simulink model "simulAMR_stateflow_indoor"  (R2024a)
settings: Solver=ode1  StartTime=0.0  StopTime=tfinal  FixedStep=tstep  MaxStep=tstep  RelTol=1e-3
values from neighbouring files (symbols this model uses):
  vehicle_wheelbase = 1    [TricycleModel.m]
undefined symbols (not defined in the file or in its folder): L, num_of_wps, T, tstep
libraries: simulink_extras x2, simulink x2
settings Model: Creator=ander  LastModifiedBy=matlab.cut

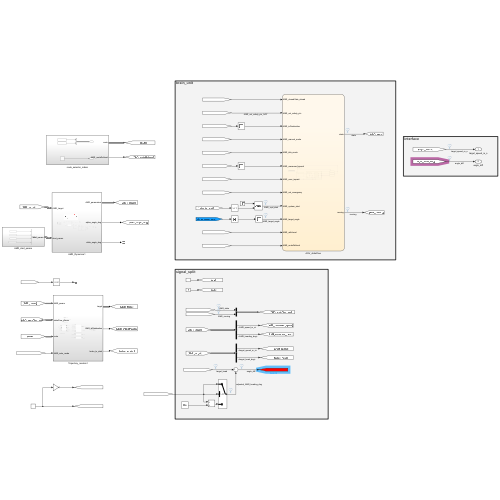
[thumbnail: Simulink's stored preview of the top-level diagram]
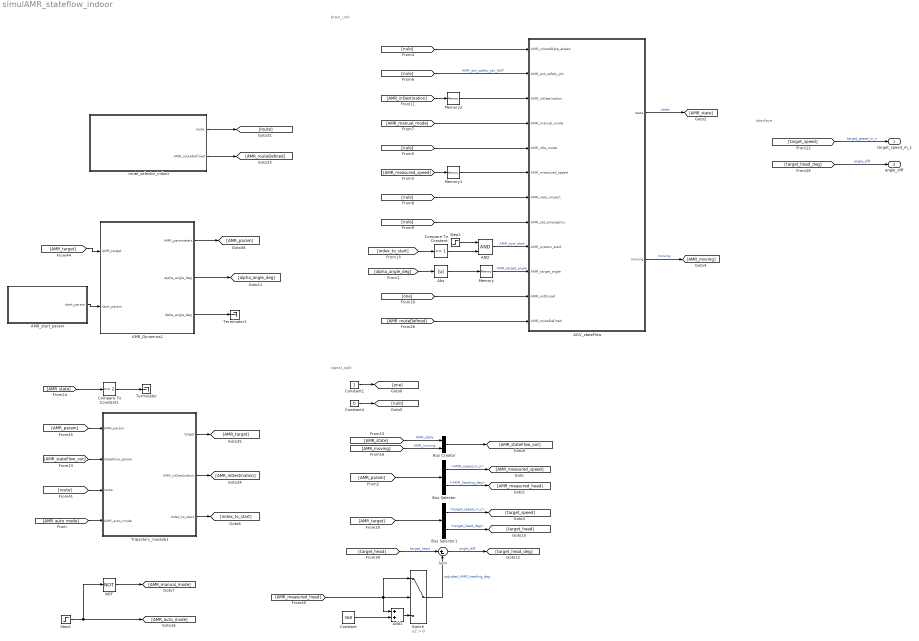
== system simulAMR_stateflow_indoor ==
  note: brain_unit
  note: interface
  note: signal_split
  AGV_stateFlow : Stateflow chart  TreatAsAtomicUnit=on
  AMR_Dynamics1 : Subsystem
  AMR_start_param : Subsystem
  AND : Logic  AllPortsSameDT=off  OutDataTypeStr=boolean
  Abs : Abs  SaturateOnIntegerOverflow=off
  Add1 : Sum
  Bus Creator : BusCreator  Inputs=2
  Bus Selector : BusSelector  OutputSignals=AMR_speed_m_s,AMR_heading_deg
  Bus Selector1 : BusSelector  OutputSignals=target_speed_m_s,target_head_deg
  Compare To Constant : simulink/Logic and Bit Operations/Compare To Constant  relop=>=  const=1  OutDataTypeStr=boolean
  Compare To Constant1 : simulink/Logic and Bit Operations/Compare To Constant  relop===  const=2  OutDataTypeStr=boolean
  Constant : Constant  Value=360
  Constant1 : Constant
  Constant4 : Constant  Value=0
  Memory : Memory
  Memory1 : Memory
  Memory2 : Memory
  NOT : Logic  Operator=NOT  IconShape=distinctive  AllPortsSameDT=off  OutDataTypeStr=boolean
  Step1 : Step  Time=20  SampleTime=tstep
  Step2 : Step  Time=10  SampleTime=0
  Sum : Sum  Inputs=|+-
  Switch : Switch  Criteria=u2 > Threshold  SaturateOnIntegerOverflow=off  InputSameDT=off
  Terminator : Terminator
  Terminator1 : Terminator
  Trajectory_module1 : Subsystem
  route_selector_indoor : Subsystem
  target_speed_m_s : Outport
  angle_diff : Outport  Port=2
  wires:
  Trajectory_module1/1(target) -> [AMR_target]
  route_selector_indoor/1(route) -> [route]
  [AMR_param] -> Trajectory_module1/1(AMR_param)
  [AMR_routeDefined] -> AGV_stateFlow/12(AMR_routeDefined)
  [nulo] -> AGV_stateFlow/1(AMR_closedGate_ahead)
  AGV_stateFlow/2(moving) -> [AMR_moving]  "moving"
  [nulo] -> AGV_stateFlow/2(AMR_ext_safety_plc)  "AMR_ext_safety_plc_NOT"
  Memory/1 -> AGV_stateFlow/10(AMR_target_angle)  "AMR_target_angle"
  Memory1/1 -> AGV_stateFlow/6(AMR_measured_speed)
  Memory2/1 -> AGV_stateFlow/3(AMR_inDestination)
  [nulo] -> AGV_stateFlow/7(AMR_near_impact)
  AGV_stateFlow/1(state) -> [AMR_state]  "state"
  [AMR_measured_speed] -> Memory1/1
  [AMR_inDestination] -> Memory2/1
  route_selector_indoor/2(AMR_routeDefined) -> [AMR_routeDefined]
  Trajectory_module1/2(AMR_inDestination) -> [AMR_inDestination]
  AMR_Dynamics1/1(AMR_parameters) -> [AMR_param]
  [one] -> AGV_stateFlow/11(AMR_withLoad)
  [AMR_stateFlow_out] -> Trajectory_module1/2(stateFlow_param)
  [AMR_manual_mode] -> AGV_stateFlow/4(AMR_manual_mode)
  [target_head_deg] -> angle_diff/1  "angle_diff"
  [route] -> Trajectory_module1/3(route)
  [nulo] -> AGV_stateFlow/5(AMR_idle_mode)
  [AMR_state] -> Compare To Constant1/1
  [AMR_target] -> AMR_Dynamics1/1(AMR_target)
  [alpha_angle_deg] -> Abs/1
  AMR_start_param/1(start_param) -> AMR_Dynamics1/2(start_param)
  [target_speed] -> target_speed_m_s/1  "target_speed_m_s"
  [target_head] -> Sum/1  "target_head"
  Switch/1 -> Sum/2  "adjusted_AMR_heading_deg"
  Constant4/1 -> [nulo]
  [AMR_param] -> Bus Selector/1
  Bus Selector1/2 -> [target_head]  "<target_head_deg>"
  Bus Selector/2 -> [AMR_measured_head]  "<AMR_heading_deg>"
  Bus Selector1/1 -> [target_speed]  "<target_speed_m_s>"
  [AMR_target] -> Bus Selector1/1
  Constant1/1 -> [one]
  [AMR_moving] -> Bus Creator/2  "AMR_moving"
  Bus Selector/1 -> [AMR_measured_speed]  "<AMR_speed_m_s>"
  [AMR_state] -> Bus Creator/1  "AMR_state"
  Bus Creator/1 -> [AMR_stateFlow_out]
  [nulo] -> AGV_stateFlow/8(AMR_set_emergency)
  Abs/1 -> Memory/1
  Step1/1 -> NOT/1, [AMR_auto_mode]
  NOT/1 -> [AMR_manual_mode]
  [AMR_auto_mode] -> Trajectory_module1/4(AMR_auto_mode)
  Compare To Constant1/1 -> Terminator/1
  Trajectory_module1/3(Index_to_start) -> [index_to_start]
  Step2/1 -> AND/1
  [index_to_start] -> Compare To Constant/1
  AND/1 -> AGV_stateFlow/9(AMR_system_start)  "AMR_syst_start"
  Compare To Constant/1 -> AND/2
  Sum/1 -> [target_head_deg]  "angle_diff"
  [AMR_measured_head] -> Switch/1, Add1/1, Switch/2
  Constant/1 -> Add1/2
  Add1/1 -> Switch/3
  AMR_Dynamics1/2(alpha_angle_deg) -> [alpha_angle_deg]
  AMR_Dynamics1/3(delta_angle_deg) -> Terminator1/1

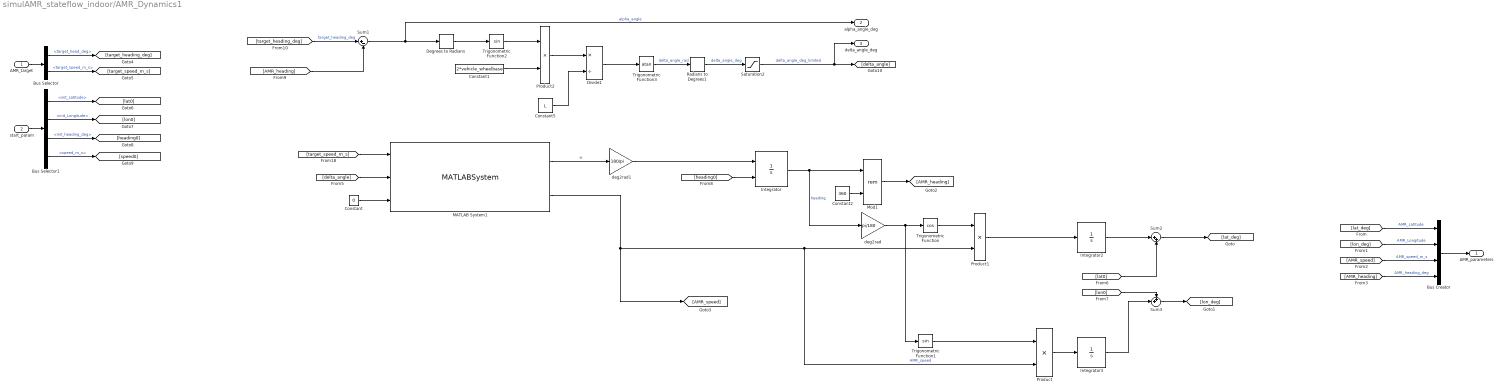
== system simulAMR_stateflow_indoor/AMR_Dynamics1 ==
  AMR_target : Inport
  start_param : Inport  Port=2
  Bus Creator : BusCreator  Inputs=4
  Bus Selector : BusSelector  OutputSignals=target_head_deg,target_speed_m_s
  Bus Selector1 : BusSelector  OutputSignals=init_Latitude,init_Longitude,init_heading_deg,speed_m_s
  Constant : Constant  Value=0
  Constant1 : Constant  Value=2*vehicle_wheelbase
  Constant2 : Constant  Value=360
  Constant5 : Constant  Value=L
  Degrees to Radians : simulink_extras/Transformations/Degrees to Radians
  Divide1 : Product  Inputs=*/
  Integrator : Integrator  InitialConditionSource=external  UpperSaturationLimit=360  LowerSaturationLimit=0
  Integrator2 : Integrator
  Integrator3 : Integrator
  MATLAB System1 : MATLABSystem  System=TricycleModel  wheel_radius=0.18  vehicle_track=0.877  vehicle_wheelbase=2.367  x0=0  y0=0  theta0=0  steering_wheel_radius=0.18  SimulateUsing=Code generation
      mask Type: TricycleModel
      mask Display:
      | disp('TricycleModel');
      | port_label('input',1,'front_wheel_speed');
      | port_label('input',2,'steering_angle');
      | port_label('input',3,'x0');
      | port_label('output',1,'angular_speed');
      | port_label('output',2,'speed');
  Mod1 : Math  Operator=rem
  Product : Product
  Product1 : Product
  Product2 : Product
  Radians to Degrees1 : simulink_extras/Transformations/Radians to Degrees
  Saturation2 : Saturate  UpperLimit=60  LowerLimit=-60
  Sum1 : Sum  Inputs=|+-
  Sum2 : Sum  Inputs=|++
  Sum3 : Sum  Inputs=++|
  Trigonometric Function : Trigonometry  Operator=cos
  Trigonometric Function1 : Trigonometry
  Trigonometric Function2 : Trigonometry
  Trigonometric Function3 : Trigonometry  Operator=atan  ApproximationMethod=CORDIC
  deg2rad : Gain  Gain=pi/180
  deg2rad1 : Gain  Gain=180/pi
  AMR_parameters : Outport
  alpha_angle_deg : Outport  Port=2
  delta_angle_deg : Outport  Port=3
  wires:
  Integrator/1 -> Mod1/1, deg2rad/1  "heading"
  MATLAB System1/2 -> [AMR_speed], Product1/2, Product/2  "AMR_speed"
  [heading0] -> Integrator/2
  deg2rad/1 -> Trigonometric Function1/1, Trigonometric Function/1
  Trigonometric Function/1 -> Product1/1
  Product1/1 -> Integrator2/1
  [lat_deg] -> Bus Creator/1  "AMR_Latitude"
  [lon_deg] -> Bus Creator/2  "AMR_Longitude"
  Bus Creator/1 -> AMR_parameters/1
  [AMR_speed] -> Bus Creator/3  "AMR_speed_m_s"
  [AMR_heading] -> Bus Creator/4  "AMR_heading_deg"
  AMR_target/1 -> Bus Selector/1
  start_param/1 -> Bus Selector1/1
  Bus Selector/1 -> [target_heading_deg]  "<target_head_deg>"
  Bus Selector/2 -> [target_speed_m_s]  "<target_speed_m_s>"
  Bus Selector1/1 -> [lat0]  "<init_Latitude>"
  Bus Selector1/2 -> [lon0]  "<init_Longitude>"
  Bus Selector1/3 -> [heading0]  "<init_heading_deg>"
  Bus Selector1/4 -> [speed0]  "<speed_m_s>"
  Product/1 -> Integrator3/1
  Trigonometric Function1/1 -> Product/1
  Sum2/1 -> [lat_deg]
  Sum3/1 -> [lon_deg]
  [lon0] -> Sum3/1
  Integrator3/1 -> Sum3/2
  MATLAB System1/1 -> deg2rad1/1  "w"
  Constant2/1 -> Mod1/2
  Mod1/1 -> [AMR_heading]
  Integrator2/1 -> Sum2/1
  [lat0] -> Sum2/2
  [target_speed_m_s] -> MATLAB System1/1
  Constant/1 -> MATLAB System1/3
  [delta_angle] -> MATLAB System1/2
  deg2rad1/1 -> Integrator/1
  [AMR_heading] -> Sum1/2
  Degrees to Radians/1 -> Trigonometric Function2/1
  Trigonometric Function2/1 -> Product2/1
  [target_heading_deg] -> Sum1/1  "target_heading_deg"
  Divide1/1 -> Trigonometric Function3/1
  Trigonometric Function3/1 -> Radians to Degrees1/1  "delta_angle_rad"
  Constant5/1 -> Divide1/2
  Product2/1 -> Divide1/1
  Constant1/1 -> Product2/2
  Sum1/1 -> alpha_angle_deg/1, Degrees to Radians/1  "alpha_angle"
  Radians to Degrees1/1 -> Saturation2/1  "delta_angle_deg"
  Saturation2/1 -> delta_angle_deg/1, [delta_angle]  "delta_angle_deg_limited"

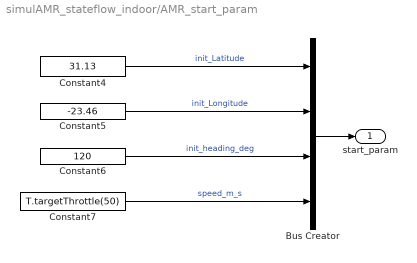
== system simulAMR_stateflow_indoor/AMR_start_param ==
  Bus Creator : BusCreator  Inputs=4
  Constant4 : Constant  Value=31.13
  Constant5 : Constant  Value=-23.46
  Constant6 : Constant  Value=120
  Constant7 : Constant  Value=T.targetThrottle(50)  VectorParams1D=off
  start_param : Outport
  wires:
  Bus Creator/1 -> start_param/1
  Constant4/1 -> Bus Creator/1  "init_Latitude"
  Constant5/1 -> Bus Creator/2  "init_Longitude"
  Constant6/1 -> Bus Creator/3  "init_heading_deg"
  Constant7/1 -> Bus Creator/4  "speed_m_s"

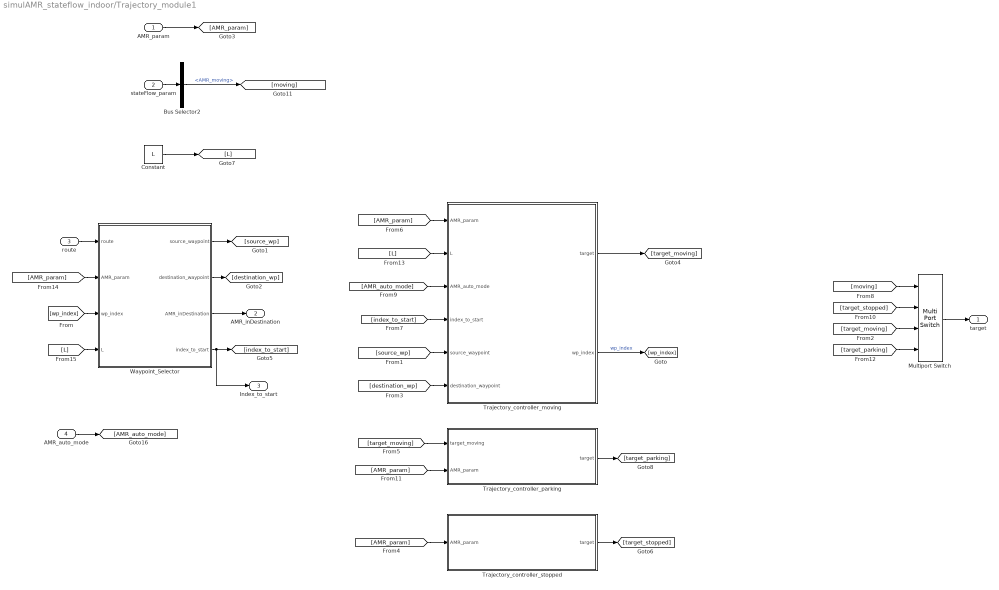
== system simulAMR_stateflow_indoor/Trajectory_module1 ==
  AMR_param : Inport
  stateFlow_param : Inport  Port=2
  route : Inport  Port=3
  AMR_auto_mode : Inport  Port=4
  Bus Selector2 : BusSelector  OutputSignals=AMR_moving
  Constant : Constant  Value=L
  Multiport Switch : MultiPortSwitch  DataPortOrder=Zero-based contiguous  zeroidx=on  SaturateOnIntegerOverflow=off  InputSameDT=off
  Trajectory_controller_moving : Subsystem
  Trajectory_controller_parking : Subsystem
  Trajectory_controller_stopped : Subsystem
  Waypoint_Selector : Subsystem
  target : Outport
  AMR_inDestination : Outport  Port=2
  Index_to_start : Outport  Port=3
  wires:
  Trajectory_controller_moving/2(wp_index) -> [wp_index]  "wp_index"
  [wp_index] -> Waypoint_Selector/3(wp_index)
  Trajectory_controller_moving/1(target) -> [target_moving]
  route/1 -> Waypoint_Selector/1(route)
  [L] -> Trajectory_controller_moving/2(L)
  Bus Selector2/1 -> [moving]  "<AMR_moving>"
  stateFlow_param/1 -> Bus Selector2/1
  [source_wp] -> Trajectory_controller_moving/5(source_waypoint)
  Waypoint_Selector/1(source_waypoint) -> [source_wp]
  Waypoint_Selector/2(destination_waypoint) -> [destination_wp]
  [destination_wp] -> Trajectory_controller_moving/6(destination_waypoint)
  AMR_param/1 -> [AMR_param]
  [AMR_param] -> Trajectory_controller_moving/1(AMR_param)
  Multiport Switch/1 -> target/1
  [moving] -> Multiport Switch/1
  [target_stopped] -> Multiport Switch/2
  [target_moving] -> Trajectory_controller_parking/1(target_moving)
  Trajectory_controller_parking/1(target) -> [target_parking]
  [AMR_param] -> Trajectory_controller_parking/2(AMR_param)
  [AMR_param] -> Trajectory_controller_stopped/1(AMR_param)
  Trajectory_controller_stopped/1(target) -> [target_stopped]
  Constant/1 -> [L]
  [AMR_param] -> Waypoint_Selector/2(AMR_param)
  [L] -> Waypoint_Selector/4(L)
  Waypoint_Selector/3(AMR_inDestination) -> AMR_inDestination/1
  [target_moving] -> Multiport Switch/3
  [target_parking] -> Multiport Switch/4
  Waypoint_Selector/4(index_to_start) -> Index_to_start/1, [index_to_start]
  [index_to_start] -> Trajectory_controller_moving/4(index_to_start)
  AMR_auto_mode/1 -> [AMR_auto_mode]
  [AMR_auto_mode] -> Trajectory_controller_moving/3(AMR_auto_mode)

== system simulAMR_stateflow_indoor/route_selector_indoor ==
  Bus Creator : BusCreator  Inputs=2
  Constant : Constant  Value=T.X
  Constant1 : Constant  Value=T.Y
  Constant2 : Constant
  route : Outport
  AMR_routeDefined : Outport  Port=2
  wires:
  Constant1/1 -> Bus Creator/2  "Y"
  Constant/1 -> Bus Creator/1  "X"
  Bus Creator/1 -> route/1  "route"
  Constant2/1 -> AMR_routeDefined/1

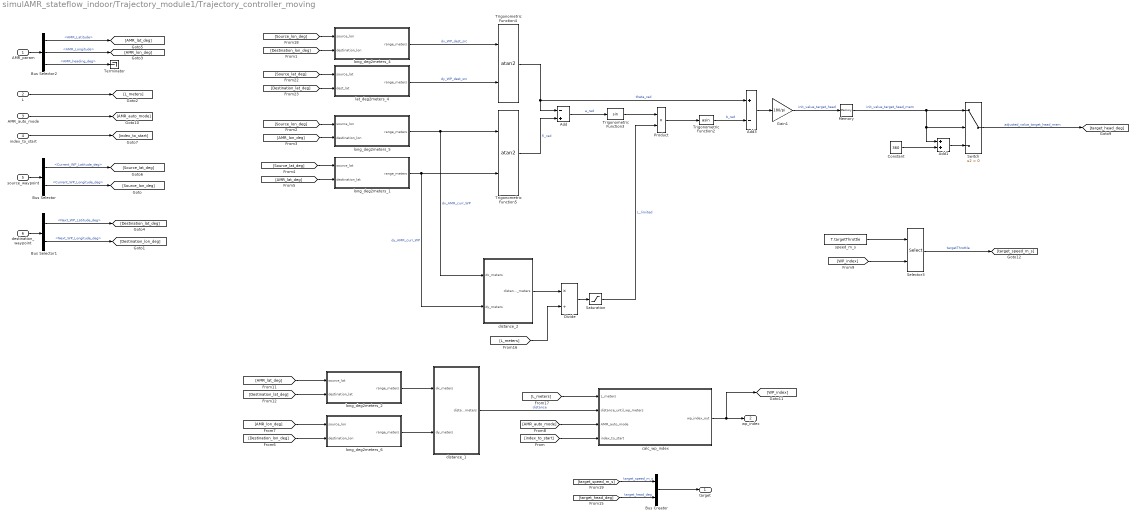
== system simulAMR_stateflow_indoor/Trajectory_module1/Trajectory_controller_moving ==
  AMR_param : Inport
  L : Inport  Port=2
  AMR_auto_mode : Inport  Port=3
  index_to_start : Inport  Port=4
  source_waypoint : Inport  Port=5
  destination_waypoint : Inport  Port=6
  Add : Sum  Inputs=-+
  Add1 : Sum
  Add3 : Sum  Inputs=+-
  Bus Creator : BusCreator  Inputs=2
  Bus Selector : BusSelector  OutputSignals=Current_WP_Latitude_deg,Current_WP_Longitude_deg
  Bus Selector1 : BusSelector  OutputSignals=Next_WP_Latitude_deg,Next_WP_Longitude_deg
  Bus Selector2 : BusSelector  OutputSignals=AMR_Latitude,AMR_Longitude,AMR_heading_deg
  Constant : Constant  Value=360
  Divide : Product  Inputs=*/
  Gain1 : Gain  Gain=180/pi
  Memory : Memory  InitialCondition=T.Yaw(1)
  Product : Product
  Saturation : Saturate  LowerLimit=0
  Selector3 : Selector  InputPortWidth=num_of_wps  IndexOptions=Index vector (port)  Indices=[1 3]  OutputSizes=1
  Switch : Switch  Criteria=u2 > Threshold  SaturateOnIntegerOverflow=off  InputSameDT=off
  Terminator : Terminator
  Trigonometric Function2 : Trigonometry  Operator=asin
  Trigonometric Function3 : Trigonometry
  Trigonometric Function4 : Trigonometry  Operator=atan2
  Trigonometric Function5 : Trigonometry  Operator=atan2
  calc_wp_index : Subsystem
  distance_1 : Subsystem  TreatAsAtomicUnit=on
  distance_2 : Subsystem  TreatAsAtomicUnit=on
  lat_deg2meters_4 : Subsystem  TreatAsAtomicUnit=on
  long_deg2meters_1 : Subsystem  TreatAsAtomicUnit=on
  long_deg2meters_2 : Subsystem  TreatAsAtomicUnit=on
  long_deg2meters_4 : Subsystem  TreatAsAtomicUnit=on
  long_deg2meters_5 : Subsystem  TreatAsAtomicUnit=on
  long_deg2meters_6 : Subsystem  TreatAsAtomicUnit=on
  speed_m_s : Constant  Value=T.targetThrottle
  target : Outport
  wp_index : Outport  Port=2
  wires:
  distance_1/1(distance_meters) -> calc_wp_index/2(distance_until_wp_meters)  "distance"
  calc_wp_index/1(wp_index_out) -> [WP_index], wp_index/1
  [Destination_lon_deg] -> long_deg2meters_6/2(destination_lon)
  Trigonometric Function4/1 -> Add3/1, Add/1  "theta_rad"
  [L_meters] -> Divide/2
  [L_meters] -> calc_wp_index/1(L_meters)
  source_waypoint/1 -> Bus Selector/1
  destination_waypoint/1 -> Bus Selector1/1
  AMR_param/1 -> Bus Selector2/1
  Bus Selector2/1 -> [AMR_lat_deg]  "<AMR_Latitude>"
  Bus Selector2/2 -> [AMR_lon_deg]  "<AMR_Longitude>"
  Bus Selector/1 -> [Source_lat_deg]  "<Current_WP_Latitude_deg>"
  Bus Selector1/2 -> [Destination_lon_deg]  "<Next_WP_Longitude_deg>"
  Bus Selector1/1 -> [Destination_lat_deg]  "<Next_WP_Latitude_deg>"
  Bus Selector/2 -> [Source_lon_deg]  "<Current_WP_Longitude_deg>"
  [AMR_lon_deg] -> long_deg2meters_6/1(source_lon)
  L/1 -> [L_meters]
  [target_speed_m_s] -> Bus Creator/1  "target_speed_m_s"
  [target_head_deg] -> Bus Creator/2  "target_head_deg"
  Bus Creator/1 -> target/1
  Add/1 -> Trigonometric Function3/1  "a_rad"
  Trigonometric Function3/1 -> Product/1
  Bus Selector2/3 -> Terminator/1  "<AMR_heading_deg>"
  Gain1/1 -> Memory/1  "init_value_target_head"
  distance_2/1(distance_meters) -> Divide/1
  [Destination_lat_deg] -> long_deg2meters_2/2(destination_lat)
  [AMR_lat_deg] -> long_deg2meters_2/1(source_lat)
  Trigonometric Function5/1 -> Add/2  "fi_rad"
  long_deg2meters_2/1(range_meters) -> distance_1/1(dx_meters)
  long_deg2meters_6/1(range_meters) -> distance_1/2(dy_meters)
  long_deg2meters_4/1(range_meters) -> Trigonometric Function4/1  "dx_WP_dest_src"
  lat_deg2meters_4/1(range_meters) -> Trigonometric Function4/2  "dy_WP_dest_src"
  long_deg2meters_5/1(range_meters) -> Trigonometric Function5/1, distance_2/1(dx_meters)  "dx_AMR_curr_WP"
  long_deg2meters_1/1(range_meters) -> Trigonometric Function5/2, distance_2/2(dy_meters)  "dy_AMR_curr_WP"
  Add3/1 -> Gain1/1
  [Source_lon_deg] -> long_deg2meters_5/1(source_lon)
  [Source_lat_deg] -> lat_deg2meters_4/1(source_lat)
  [Destination_lon_deg] -> long_deg2meters_4/2(destination_lon)
  [AMR_lon_deg] -> long_deg2meters_5/2(destination_lon)
  [Destination_lat_deg] -> lat_deg2meters_4/2(dest_lat)
  [Source_lon_deg] -> long_deg2meters_4/1(source_lon)
  Trigonometric Function2/1 -> Add3/2  "b_rad"
  Product/1 -> Trigonometric Function2/1
  Divide/1 -> Saturation/1
  Saturation/1 -> Product/2  "L_limited"
  [Source_lat_deg] -> long_deg2meters_1/1(source_lat)
  [AMR_lat_deg] -> long_deg2meters_1/2(destination_lat)
  Memory/1 -> Add1/1, Switch/2, Switch/1  "init_value_target_head_mem"
  index_to_start/1 -> [index_to_start]
  [index_to_start] -> calc_wp_index/4(index_to_start)
  [AMR_auto_mode] -> calc_wp_index/3(AMR_auto_mode)
  AMR_auto_mode/1 -> [AMR_auto_mode]
  speed_m_s/1 -> Selector3/1
  [WP_index] -> Selector3/2
  Selector3/1 -> [target_speed_m_s]  "targetThrottle"
  Switch/1 -> [target_head_deg]  "adjusted_value_target_head_mem"
  Add1/1 -> Switch/3
  Constant/1 -> Add1/2

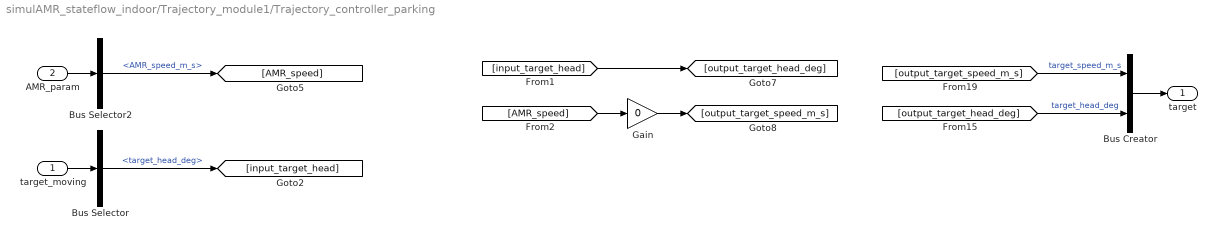
== system simulAMR_stateflow_indoor/Trajectory_module1/Trajectory_controller_parking ==
  target_moving : Inport
  AMR_param : Inport  Port=2
  Bus Creator : BusCreator  Inputs=2
  Bus Selector : BusSelector  OutputSignals=target_head_deg
  Bus Selector2 : BusSelector  OutputSignals=AMR_speed_m_s
  Gain : Gain  Gain=0
  target : Outport
  wires:
  [output_target_speed_m_s] -> Bus Creator/1  "target_speed_m_s"
  [output_target_head_deg] -> Bus Creator/2  "target_head_deg"
  Bus Creator/1 -> target/1
  [input_target_head] -> [output_target_head_deg]
  target_moving/1 -> Bus Selector/1
  AMR_param/1 -> Bus Selector2/1
  Bus Selector2/1 -> [AMR_speed]  "<AMR_speed_m_s>"
  Bus Selector/1 -> [input_target_head]  "<target_head_deg>"
  Gain/1 -> [output_target_speed_m_s]
  [AMR_speed] -> Gain/1

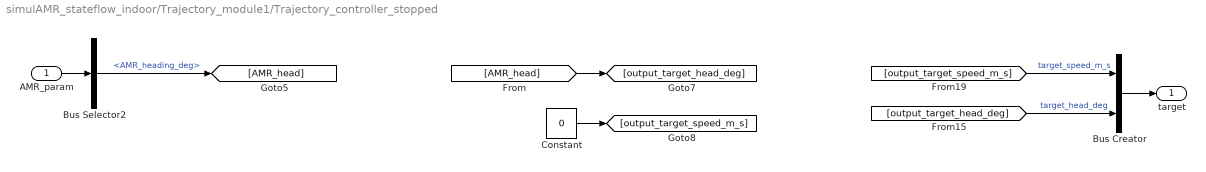
== system simulAMR_stateflow_indoor/Trajectory_module1/Trajectory_controller_stopped ==
  AMR_param : Inport
  Bus Creator : BusCreator  Inputs=2
  Bus Selector2 : BusSelector  OutputSignals=AMR_heading_deg
  Constant : Constant  Value=0
  target : Outport
  wires:
  [output_target_speed_m_s] -> Bus Creator/1  "target_speed_m_s"
  [output_target_head_deg] -> Bus Creator/2  "target_head_deg"
  Bus Creator/1 -> target/1
  [AMR_head] -> [output_target_head_deg]
  AMR_param/1 -> Bus Selector2/1
  Bus Selector2/1 -> [AMR_head]  "<AMR_heading_deg>"
  Constant/1 -> [output_target_speed_m_s]

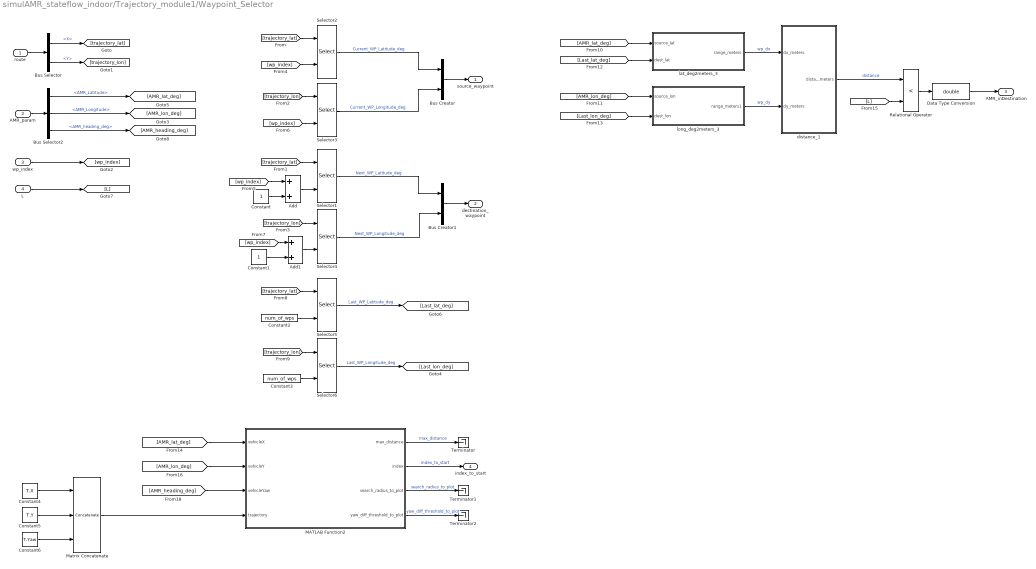
== system simulAMR_stateflow_indoor/Trajectory_module1/Waypoint_Selector ==
  route : Inport
  AMR_param : Inport  Port=2
  wp_index : Inport  Port=3
  L : Inport  Port=4
  Add : Sum
  Add1 : Sum
  Bus Creator : BusCreator  Inputs=2
  Bus Creator1 : BusCreator  Inputs=2
  Bus Selector : BusSelector  OutputSignals=X,Y
  Bus Selector2 : BusSelector  OutputSignals=AMR_Latitude,AMR_Longitude,AMR_heading_deg
  Constant : Constant
  Constant1 : Constant
  Constant2 : Constant  Value=num_of_wps
  Constant3 : Constant  Value=num_of_wps
  Constant4 : Constant  Value=T.X
  Constant5 : Constant  Value=T.Y
  Constant6 : Constant  Value=T.Yaw
  Data Type Conversion : DataTypeConversion  OutDataTypeStr=double  SaturateOnIntegerOverflow=off  RndMeth=Floor
  MATLAB Function2 : MATLAB Function  TreatAsAtomicUnit=on
  Matrix Concatenate : Concatenate  NumInputs=3  Mode=Multidimensional array  ConcatenateDimension=2
  Relational Operator : RelationalOperator  Operator=<  OutDataTypeStr=boolean  RndMeth=Simplest  InputSameDT=off
  Selector{1..6} (6 alike) : Selector  InputPortWidth=num_of_wps  IndexOptions=Index vector (port)  Indices=[1 3]  OutputSizes=1
  Terminator : Terminator
  Terminator1 : Terminator
  Terminator2 : Terminator
  distance_1 : Subsystem  TreatAsAtomicUnit=on
  lat_deg2meters_3 : Subsystem  TreatAsAtomicUnit=on
  long_deg2meters_3 : Subsystem  TreatAsAtomicUnit=on
  source_waypoint : Outport
  destination_waypoint : Outport  Port=2
  AMR_inDestination : Outport  Port=3
  index_to_start : Outport  Port=4
  wires:
  Selector2/1 -> Bus Creator/1  "Current_WP_Latitude_deg"
  Add/1 -> Selector1/2
  Constant/1 -> Add/2
  Constant1/1 -> Add1/2
  Add1/1 -> Selector4/2
  route/1 -> Bus Selector/1
  Bus Selector/1 -> [trajectory_lat]  "<X>"
  Bus Selector/2 -> [trajectory_lon]  "<Y>"
  [trajectory_lat] -> Selector2/1
  [trajectory_lat] -> Selector1/1
  [trajectory_lon] -> Selector3/1
  [trajectory_lon] -> Selector4/1
  wp_index/1 -> [wp_index]
  [wp_index] -> Selector2/2
  [wp_index] -> Add/1
  [wp_index] -> Selector3/2
  [wp_index] -> Add1/1
  Bus Creator/1 -> source_waypoint/1
  Selector3/1 -> Bus Creator/2  "Current_WP_Longitude_deg"
  Selector4/1 -> Bus Creator1/2  "Next_WP_Longitude_deg"
  Selector1/1 -> Bus Creator1/1  "Next_WP_Latitude_deg"
  Bus Creator1/1 -> destination_waypoint/1
  Bus Selector2/1 -> [AMR_lat_deg]  "<AMR_Latitude>"
  AMR_param/1 -> Bus Selector2/1
  Bus Selector2/2 -> [AMR_lon_deg]  "<AMR_Longitude>"
  [trajectory_lat] -> Selector5/1
  [trajectory_lon] -> Selector6/1
  Constant3/1 -> Selector6/2
  Constant2/1 -> Selector5/2
  long_deg2meters_3/1(range_meters1) -> distance_1/2(dy_meters)  "wp_dy"
  lat_deg2meters_3/1(range_meters) -> distance_1/1(dx_meters)  "wp_dx"
  Selector5/1 -> [Last_lat_deg]  "Last_WP_Latitude_deg"
  Selector6/1 -> [Last_lon_deg]  "Last_WP_Longitude_deg"
  [AMR_lat_deg] -> lat_deg2meters_3/1(source_lat)
  Relational Operator/1 -> Data Type Conversion/1
  distance_1/1(distance_meters) -> Relational Operator/1  "distance"
  L/1 -> [L]
  [L] -> Relational Operator/2
  Data Type Conversion/1 -> AMR_inDestination/1
  [Last_lat_deg] -> lat_deg2meters_3/2(dest_lat)
  [AMR_lon_deg] -> long_deg2meters_3/1(source_lon)
  [Last_lon_deg] -> long_deg2meters_3/2(dest_lon)
  [AMR_lat_deg] -> MATLAB Function2/1(vehicleX)
  [AMR_lon_deg] -> MATLAB Function2/2(vehicleY)
  Constant6/1 -> Matrix Concatenate/3
  Constant4/1 -> Matrix Concatenate/1
  Constant5/1 -> Matrix Concatenate/2
  Matrix Concatenate/1 -> MATLAB Function2/4(trajectory)
  [AMR_heading_deg] -> MATLAB Function2/3(vehicleYaw)
  Bus Selector2/3 -> [AMR_heading_deg]  "<AMR_heading_deg>"
  MATLAB Function2/3(search_radius_to_plot) -> Terminator1/1  "search_radius_to_plot"
  MATLAB Function2/4(yaw_diff_threshold_to_plot) -> Terminator2/1  "yaw_diff_threshold_to_plot"
  MATLAB Function2/2(index) -> index_to_start/1  "index_to_start"
  MATLAB Function2/1(max_distance) -> Terminator/1  "max_distance"

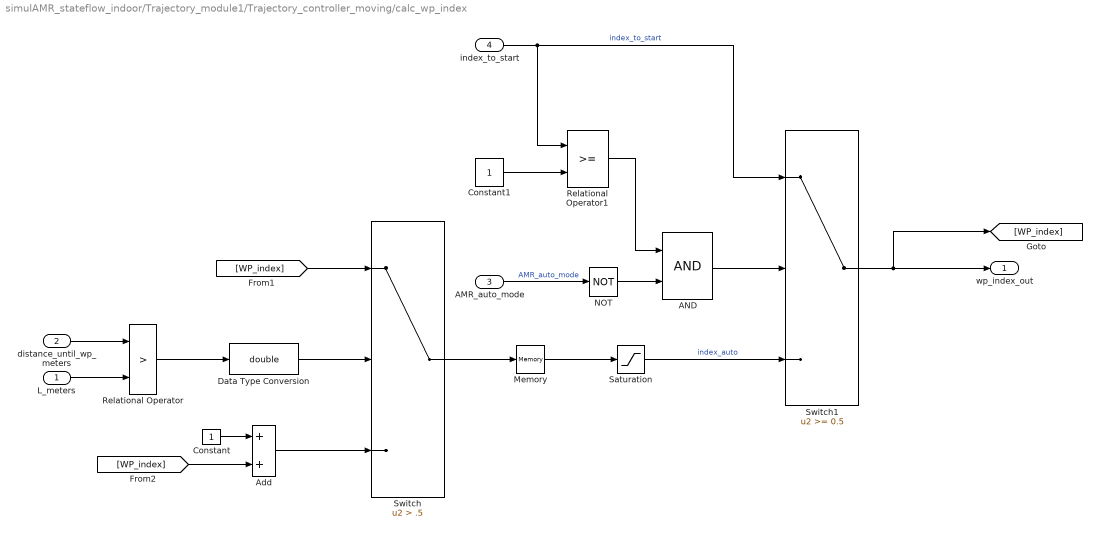
== system simulAMR_stateflow_indoor/Trajectory_module1/Trajectory_controller_moving/calc_wp_index ==
  L_meters : Inport
  distance_until_wp_meters : Inport  Port=2
  AMR_auto_mode : Inport  Port=3
  index_to_start : Inport  Port=4
  AND : Logic  AllPortsSameDT=off  OutDataTypeStr=boolean
  Add : Sum
  Constant : Constant
  Constant1 : Constant
  Data Type Conversion : DataTypeConversion  OutDataTypeStr=double  SaturateOnIntegerOverflow=off  RndMeth=Floor
  Memory : Memory  InitialCondition=1
  NOT : Logic  Operator=NOT  IconShape=distinctive  AllPortsSameDT=off  OutDataTypeStr=boolean
  Relational Operator : RelationalOperator  Operator=>  OutDataTypeStr=boolean  RndMeth=Simplest  InputSameDT=off
  Relational Operator1 : RelationalOperator  OutDataTypeStr=boolean  RndMeth=Simplest  InputSameDT=off
  Saturation : Saturate  UpperLimit=num_of_wps-1  LowerLimit=1
  Switch : Switch  Criteria=u2 > Threshold  Threshold=.5  SaturateOnIntegerOverflow=off  InputSameDT=off
  Switch1 : Switch  Threshold=0.5  SaturateOnIntegerOverflow=off  InputSameDT=off
  wp_index_out : Outport
  wires:
  distance_until_wp_meters/1 -> Relational Operator/1
  L_meters/1 -> Relational Operator/2
  Relational Operator/1 -> Data Type Conversion/1
  Data Type Conversion/1 -> Switch/2
  Switch/1 -> Memory/1
  Add/1 -> Switch/3
  Constant/1 -> Add/1
  [WP_index] -> Switch/1
  [WP_index] -> Add/2
  Memory/1 -> Saturation/1
  Switch1/1 -> [WP_index], wp_index_out/1
  Saturation/1 -> Switch1/3  "index_auto"
  index_to_start/1 -> Switch1/1, Relational Operator1/1  "index_to_start"
  Constant1/1 -> Relational Operator1/2
  Relational Operator1/1 -> AND/1
  AMR_auto_mode/1 -> NOT/1  "AMR_auto_mode"
  AND/1 -> Switch1/2
  NOT/1 -> AND/2

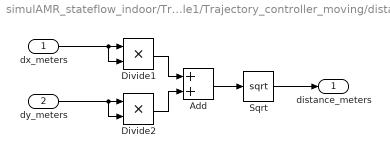
== system simulAMR_stateflow_indoor/Trajectory_module1/Trajectory_controller_moving/distance_1 ==
  dx_meters : Inport
  dy_meters : Inport  Port=2
  Add : Sum
  Divide1 : Product  Inputs=**
  Divide2 : Product  Inputs=**
  Sqrt : Sqrt
  distance_meters : Outport
  wires:
  dx_meters/1 -> Divide1/2, Divide1/1
  Divide1/1 -> Add/1
  Add/1 -> Sqrt/1
  dy_meters/1 -> Divide2/2, Divide2/1
  Divide2/1 -> Add/2
  Sqrt/1 -> distance_meters/1

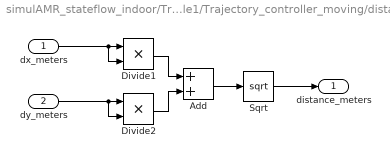
== system simulAMR_stateflow_indoor/Trajectory_module1/Trajectory_controller_moving/distance_2 ==
  dx_meters : Inport
  dy_meters : Inport  Port=2
  Add : Sum
  Divide1 : Product  Inputs=**
  Divide2 : Product  Inputs=**
  Sqrt : Sqrt
  distance_meters : Outport
  wires:
  dx_meters/1 -> Divide1/2, Divide1/1
  Divide1/1 -> Add/1
  Add/1 -> Sqrt/1
  dy_meters/1 -> Divide2/2, Divide2/1
  Divide2/1 -> Add/2
  Sqrt/1 -> distance_meters/1

== system simulAMR_stateflow_indoor/Trajectory_module1/Trajectory_controller_moving/lat_deg2meters_4 ==
  source_lat : Inport
  dest_lat : Inport  Port=2
  Add : Sum  Inputs=+-
  range_meters : Outport
  wires:
  Add/1 -> range_meters/1
  dest_lat/1 -> Add/1
  source_lat/1 -> Add/2

== system simulAMR_stateflow_indoor/Trajectory_module1/Trajectory_controller_moving/long_deg2meters_1 ==
  source_lat : Inport
  destination_lat : Inport  Port=2
  Add : Sum  Inputs=+-
  range_meters : Outport
  wires:
  source_lat/1 -> Add/2
  destination_lat/1 -> Add/1
  Add/1 -> range_meters/1

== system simulAMR_stateflow_indoor/Trajectory_module1/Trajectory_controller_moving/long_deg2meters_2 ==
  source_lat : Inport
  destination_lat : Inport  Port=2
  Add : Sum  Inputs=+-
  range_meters : Outport
  wires:
  Add/1 -> range_meters/1
  destination_lat/1 -> Add/1
  source_lat/1 -> Add/2

== system simulAMR_stateflow_indoor/Trajectory_module1/Trajectory_controller_moving/long_deg2meters_4 ==
  source_lon : Inport
  destination_lon : Inport  Port=2
  Add1 : Sum  Inputs=+-
  range_meters : Outport
  wires:
  source_lon/1 -> Add1/2
  Add1/1 -> range_meters/1
  destination_lon/1 -> Add1/1

== system simulAMR_stateflow_indoor/Trajectory_module1/Trajectory_controller_moving/long_deg2meters_5 ==
  source_lon : Inport
  destination_lon : Inport  Port=2
  Add : Sum  Inputs=+-
  range_meters : Outport
  wires:
  source_lon/1 -> Add/2
  destination_lon/1 -> Add/1
  Add/1 -> range_meters/1

== system simulAMR_stateflow_indoor/Trajectory_module1/Trajectory_controller_moving/long_deg2meters_6 ==
  source_lon : Inport
  destination_lon : Inport  Port=2
  Add : Sum  Inputs=+-
  range_meters : Outport
  wires:
  Add/1 -> range_meters/1
  destination_lon/1 -> Add/1
  source_lon/1 -> Add/2

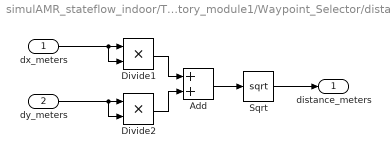
== system simulAMR_stateflow_indoor/Trajectory_module1/Waypoint_Selector/distance_1 ==
  dx_meters : Inport
  dy_meters : Inport  Port=2
  Add : Sum
  Divide1 : Product  Inputs=**
  Divide2 : Product  Inputs=**
  Sqrt : Sqrt
  distance_meters : Outport
  wires:
  dx_meters/1 -> Divide1/2, Divide1/1
  Divide1/1 -> Add/1
  Add/1 -> Sqrt/1
  dy_meters/1 -> Divide2/2, Divide2/1
  Divide2/1 -> Add/2
  Sqrt/1 -> distance_meters/1

== system simulAMR_stateflow_indoor/Trajectory_module1/Waypoint_Selector/lat_deg2meters_3 ==
  source_lat : Inport
  dest_lat : Inport  Port=2
  Add : Sum  Inputs=+-
  range_meters : Outport
  wires:
  Add/1 -> range_meters/1
  dest_lat/1 -> Add/1
  source_lat/1 -> Add/2

== system simulAMR_stateflow_indoor/Trajectory_module1/Waypoint_Selector/long_deg2meters_3 ==
  source_lon : Inport
  dest_lon : Inport  Port=2
  Add1 : Sum  Inputs=+-
  range_meters1 : Outport
  wires:
  source_lon/1 -> Add1/2
  dest_lon/1 -> Add1/1
  Add1/1 -> range_meters1/1

== matlab function simulAMR_stateflow_indoor/Trajectory_module1/Waypoint_Selector/MATLAB Function2 ==
  data: vehicleX input; vehicleY input; vehicleYaw input; trajectory input; max_distance output; index output; search_radius_to_plot output; L parameter; yaw_diff_threshold_to_plot output
function [max_distance, index, search_radius_to_plot, yaw_diff_threshold_to_plot] = findClosestTrajectoryIndex(vehicleX, vehicleY, vehicleYaw, trajectory, L)
    % Initialize variables
    max_distance = -inf;
    index = 0;
    search_radius = L;
    search_radius_to_plot = 0;
    yaw_diff_threshold_to_plot = 0; 


    while index == 0 && search_radius <= 10*L
       
       if search_radius <= 2*L
           yaw_diff_threshold = 30;
       elseif search_radius <= 5*L
           yaw_diff_threshold = 25;       
       else
           yaw_diff_threshold = 20;
       end


       for i = 1:size(trajectory, 1)-1
          % Coordinates and yaw of the line segment endpoints
          point1X = trajectory(i, 1);
          point1Y = trajectory(i, 2);
          point2X = trajectory(i+1, 1);
          point2Y = trajectory(i+1, 2);

          % Find the intersection between the line segment and a circle around the vehicle
          [x_inter, y_inter, line_segment_angle] = intersectLineCircle(point1X, point1Y, point2X, point2Y, vehicleX, vehicleY, search_radius);

          % Check if the intersection point is ahead of the vehicle
          if ~isempty(x_inter) && ~isempty(y_inter)
              vec_to_intersection = [x_inter - vehicleX, y_inter - vehicleY];
              vehicle_dir = [cosd(vehicleYaw), sind(vehicleYaw)];
              dot_product = dot(vec_to_intersection, vehicle_dir);
              
              % line segment angle
              if line_segment_angle < 0
                  line_segment_angle = line_segment_angle + 360;
              end

              % Calcula a diferença de YAW entre o veículo e o ponto atual
              vehicleYaw_to_trajectorySegmentYaw  = abs(vehicleYaw - line_segment_angle);

              % angle between the vector from the vehicle's position to the intersection point 
              intersection_angle_deg = atan2d(y_inter - vehicleY, x_inter - vehicleX);

              if intersection_angle_deg(1) < 0
                  intersection_angle_deg(1) = intersection_angle_deg(1) + 360;
              end
              
               % disp('check')
               % disp(i)
               % disp(search_radius)
               % disp(yaw_diff_threshold)
               % disp(dot_product)
               % disp(vehicleYaw)
               % disp(line_segment_angle)
               % disp(abs(vehicleYaw - intersection_angle_deg(1)))
               % disp(abs(vehicleYaw_to_trajectorySegmentYaw))

              % Check if the intersection is ahead of the vehicle and within the yaw threshold
              if dot_product(1) > 0 && ...
                      abs(vehicleYaw - intersection_angle_deg(1)) <= yaw_diff_threshold && ...
                      abs(vehicleYaw_to_trajectorySegmentYaw) <= yaw_diff_threshold 

                  distance_to_point = norm(vec_to_intersection);
                  
                  % disp('index')              
                  % disp(i)
                  % disp( vehicleYaw )
                  % disp(line_segment_angle)    
                  % disp(vec_to_intersection)
                  % disp(vehicle_dir)
                  % disp(dot_product(1) )
                  % disp('') 
                  
                  % Update the max distance and index if this point is farther away
                  if distance_to_point > max_distance
                      max_distance = distance_to_point;
                      index = i;
                      search_radius_to_plot = search_radius;
                      yaw_diff_threshold_to_plot = yaw_diff_threshold;
                  end
              end
          end
       end

       % Increase the search radius if no valid point is found
       if index == 0
           search_radius = search_radius + 0.5;
       end
    end
end




%% intersectLineCircle
function [x_inter, y_inter, line_segment_angle] = intersectLineCircle(x1, y1, x2, y2, h, k, r)
    a = (y2-y1) / (x2-x1);
    b = y1 - a*x1;
    line_segment_angle = atan2d(y2-y1,x2-x1);

    
    x_inter = [0,0];
    y_inter = [0,0];

    % Encontrar os pontos de interseção
    A = 1 + a^2;
    B = 2*(a*b - a*k - h);
    C = h^2 + b^2 + k^2 -2*b*k - r^2;

    delta = B^2 - 4*A*C;

    if delta < 0
        x_inter = [];
        y_inter = [];
        return;
    end

    x_inter(1) = (-B + sqrt(delta)) / (2*A);
    x_inter(2) = (-B - sqrt(delta)) / (2*A);

    y_inter(1) = a*x_inter(1) + b;
    y_inter(2) = a*x_inter(2) + b;
    
        
    % Verificar se os pontos de interseção estão dentro do segmento de reta
    if ((x_inter(1)-x1)*(x_inter(1)-x2) <= 0) && ((y_inter(1)-y1)*(y_inter(1)-y2) <= 0)
        % disp('pontos de interseção - ahead');
        x_inter = x_inter(1);
        y_inter = y_inter(1);
        
    elseif ((x_inter(2)-x1)*(x_inter(2)-x2) <= 0) && ((y_inter(2)-y1)*(y_inter(2)-y2) <= 0)
        % disp('pontos de interseção - behind');
        x_inter = x_inter(2);
        y_inter = y_inter(2);

    else
        x_inter = [];
        y_inter = [];
    end
end

== stateflow chart simulAMR_stateflow_indoor/AGV_stateFlow ==
  state S0_startup
    entry:
    %to_web("AGV entered boot mode (S0_startup)");
    state = 0;
    moving = 0;
    settings: description=This state models the modes of a window sensor and implements logic to respond when that sensor is producing a signal.
  state E1_failed
    entry:
    state = -1;
    moving = 0;
    %to_web("AGV failed to startup (E1_failed)!");
    settings: description=This state models the modes of a window sensor and implements logic to respond when that sensor is producing a signal.
  state autonomousOperation
    settings: description=This state models the modes of a window sensor and implements logic to respond when that sensor is producing a signal.
    state S2_engaged
      entry:
      %to_web("AGV is engaged mode (S2_engaged)");
      state = 2;
      settings: description=This state models the modes of a window sensor and implements logic to respond when that sensor is producing a signal.
      state S2A_Init
        entry:
        %to_web("AGV is rotating (S2A_Init)")
        moving = 0;
      state S2B_Moving
        entry:
        %to_web("AGV is moving (S2B_Moving)")
        moving = 1;
      state S2C_Parking
        entry:
        %to_web("AGV is slowing down (S2C_Parking)")
        moving = 2;
      state S2D_Stopped
        entry:
        %to_web("AGV is stopped (S2D_Stopped)")
        moving = 0;
      state S2E_Gate
        entry:
        %to_web("AGV is waiting gate Open (S2E_Gate)");
        moving = 0;
      (default) -> S2A_Init
      S2B_Moving -> (junction 285) [order 1] : [AMR_near_impact==TRUE]
      (junction 285) -> (junction 290)
      S2A_Init -> S2B_Moving : [AMR_target_angle <= 30]
      S2B_Moving -> S2C_Parking [order 2] : [AMR_target_angle >= 60| AMR_closedGate_ahead==TRUE | AMR_inDestination==TRUE]
      (junction 300) -> S2A_Init
      S2C_Parking -> (junction 290) [order 1] : [AMR_near_impact==TRUE]
      (junction 290) -> (junction 286)
      (junction 299) -> (junction 300)
      S2E_Gate -> (junction 300) [order 2] : [AMR_closedGate_ahead==TRUE]
      (junction 295) -> (junction 299) [order 3]
      S2C_Parking -> S2D_Stopped [order 2] : [AMR_measured_speed < 0.015]
      S2E_Gate -> S2E_Gate [order 1] : after(60, sec)
      (junction 295) -> S2E_Gate [order 2] : [AMR_closedGate_ahead==TRUE]
      S2D_Stopped -> (junction 295) : [AMR_near_impact==FALSE && AMR_measured_speed < 0.015]
      (junction 286) -> S2D_Stopped : %{to_web("AGV is near impact!");}
    state S1_standby
      entry:
      %to_web("AGV is waiting instructions (S1_standby)");
      state = 1;
      settings: description=This state models the modes of a window sensor and implements logic to respond when that sensor is producing a signal.
    state S4_unloading [commented out]
      entry:
      %to_web("AGV starting unloading process");
      state = 4;
      settings: description=This state models the modes of a window sensor and implements logic to respond when that sensor is producing a signal.
    state S3_loading [commented out]
      entry:
      %to_web("AGV starting loading process");
      state = 3;
      settings: description=This state models the modes of a window sensor and implements logic to respond when that sensor is producing a signal.
    (default) -> S1_standby
    S1_standby -> S2_engaged : [AMR_routeDefined==TRUE]
    S4_unloading -> S1_standby [commented out]
    (junction 269) -> S2_engaged [commented out]
    S3_loading -> (junction 269) [commented out]
    (junction 295) -> (junction 253) [order 1] : [AMR_inDestination==TRUE]
    (junction 333) -> S2D_Stopped
    (junction 275) -> S4_unloading [commented out]
    (junction 254) -> S3_loading [commented out] : [AGV_withLoad==FALSE]
    (junction 254) -> (junction 275) : [AMR_withLoad==TRUE]
    (junction 253) -> (junction 254) [order 1]
    (junction 253) -> (junction 333) [order 2]
  note: Constantes:
      | WAITING = 0
      | SUCCESS=1
      | FAIL=-1
      | FALSE=0
      | TRUE=1
      |
      | Flags:
      | AGV_speed_measued = double() => Captura a velocidade do AGV
      | AGV_target_angle = double() => Captura o ângulo entre o AGV e o próximo waypoing
      | AGV_near_impact = TRUE => Sensor acusa impacto iminente
      | AGV_near_impact = FALSE => Sensor de impacto diz que está livre
      | AGV_ext_safety_plc = TRUE => Estado de emergência foi resolvido
      | AGV_ext_safety_plc = FALSE => Estado de emergência não foi resolvido
      | AGV_closedGate_ahead = TRUE => Existe um portão fechado a frente
      | AGV_closedGate_ahead = FALSE => Caminho livre
      | AGV_withLoad = TRUE => AGV está com carga (segue para estado de unloading)
      | AGV_withLoad = FALSE => AGV está sem carga (segue para o estado de loading)
      | AGV_inDestination = TRUE => AGV chegou ao destino de carga ou descarga
      | AGV_inDestination = FAIL => AGV chegou ao destino de carga ou descarga
      | AGV_system_startup = WAITING => AGV não foi inicializado (aguardando)
      | AGV_system_startup = SUCCESS => AGV inicializado com sucesso
      | AGV_system_startup = FAIL => AGV inicializado com falha
      | AGV_system_emergency = TRUE => AGV vai para modo de emergência
      | AGV_system_emergency = FALSE => AGV continua sua operação normal
      | AGV_manual_mode = TRUE => AGV vai para modo manual
      | AGV_manual_mode = FALSE => AGV continua sua operação normal
      | AGV_routeDefined = TRUE => AGV com rota definida
      | AGV_routeDefined = FALSE => AGV sem rota definida
  state E2_emergency
    entry:
    state = -2;
    moving = 0;
    %fprintf("AGV está em modo de emergência!");
    settings: description=This state models the modes of a window sensor and implements logic to respond when that sensor is producing a signal.
  state E3_manualMode
    entry:
    state = -3;
    moving = 0;
    %fprintf("to web: AGV está em modo manual!\n");
    settings: description=This state models the modes of a window sensor and implements logic to respond when that sensor is producing a signal.
  (default) -> (junction 244)
  (junction 242) -> (junction 244)
  (junction 244) -> S0_startup
  (junction 312) -> (junction 242)
  S0_startup -> (junction 257) : [AMR_system_start~=WAITING]
  (junction 257) -> (junction 251) [order 1] : [AMR_system_start==FAIL]
  (junction 251) -> E1_failed
  (junction 257) -> autonomousOperation [order 2] : [AMR_system_start==SUCCESS]
  autonomousOperation -> E1_failed [order 3] : [AMR_system_start==FAIL]
  E1_failed -> (junction 312)
  (junction 243) -> (junction 312)
  E2_emergency -> (junction 243) [order 1] : [AMR_ext_safety_plc==TRUE]
  autonomousOperation -> E2_emergency [order 1] : [AMR_set_emergency==TRUE]
  E2_emergency -> E2_emergency [order 2] : after(10, sec)
  autonomousOperation -> E3_manualMode [order 2] : [AMR_manual_mode==TRUE | AMR_idle_mode==TRUE]
  E3_manualMode -> autonomousOperation : [AMR_manual_mode==FALSE | AMR_idle_mode==FALSE]
  data: msg function_input; state output =0; moving output size=1; FAIL constant double =-1; SUCCESS constant double =1; WAITING constant double =0; AMR_closedGate_ahead input; AMR_ext_safety_plc input; AMR_inDestination input; AMR_manual_mode input; AMR_idle_mode input; AMR_measured_speed input; AMR_near_impact input; AMR_set_emergency input; AMR_system_start input; AMR_target_angle input; AMR_withLoad input; FALSE constant double =0; TRUE constant double =1; AMR_routeDefined input
  function to_web(msg):
    | % Envia um log para o servidor local (em python)
    | function to_web(msg)
    |     fprintf("to web: %s\n",msg);
    |     udps = dsp.UDPSender('RemoteIPPort',31000);
    |     udps(uint8(char(msg)))
    |     release(udps)
